simulink model "HOYAS_GRANDES_I"  (R2023b)
settings: Solver=FixedStepDiscrete  StartTime=0.0  StopTime=inf  FixedStep=Ts_Power  RelTol=1e-3  EnableMultiTasking=on
PostLoadFcn:
  | Ts_Power=50e-6;f=50;R_ac=0.12;L_ac=0.08/(2*pi*50);L1=0.17874;L2=0.07596;L3=0.04321;L4=0.01471;L5=0.04751;L6=0.2054;L7=0.17263;L8=0.14418;L9=0.17697;L10=0.19944;L11=0.18905;L12=0.26987;L13=0.1671;L14=0.16874;L15=0.14664;L16=0.12477;L17=0.14989;L18=0.17217;L19=0.19436; load('PV_prof_norm.mat');
InitFcn:
  | Ts_Power=50e-6;f=50;R_ac=0.12;L_ac=0.08/(2*pi*50);L1=0.17874;L2=0.07596;L3=0.04321;L4=0.01471;L5=0.04751;L6=0.2054;L7=0.17263;L8=0.14418;L9=0.17697;L10=0.19944;L11=0.18905;L12=0.26987;L13=0.1671;L14=0.16874;L15=0.14664;L16=0.12477;L17=0.14989;L18=0.17217;L19=0.19436; load('PV_prof_norm.mat');
undefined symbols (not defined in the file or in its folder): D11, Delta, L, X_ac
libraries: spsVoltageMeasurementLib x84, spsCurrentMeasurementLib x75, rtlab x41, spsThreePhaseSeriesRLCBranchLib x38, spsGroundLib x28, powerlib_extras x25, spsThreePhaseDynamicLoadLib x19, eeGeneralControl x4, rteventslib x4, spsThreePhasePISectionLineLib x2, spsThreePhaseTransformerTwoWindingsLib x2, spsPLLLib x1
(part 4 of 4)

== system HOYAS_GRANDES_I/SM_Computation/HOYAS GRANDES CT02/HG.1_CT.2-INV.08/Subsystem1 ==
  Current Measurement : spsCurrentMeasurementLib/Current Measurement  PhasorSimulation=off  OutputType=Complex  PSBequivalent=0
  Current Measurement1 : spsCurrentMeasurementLib/Current Measurement  PhasorSimulation=off  OutputType=Complex  PSBequivalent=0
  Current Measurement2 : spsCurrentMeasurementLib/Current Measurement  PhasorSimulation=off  OutputType=Complex  PSBequivalent=0
  Mux : Mux  Inputs=3
  a : PMIOPort  Side=Right
  ia : PMIOPort  Port=2  Side=Left
  ib : PMIOPort  Port=3  Side=Left
  b : PMIOPort  Port=4  Side=Right
  ic : PMIOPort  Port=5  Side=Left
  c : PMIOPort  Port=6  Side=Right
  i : Outport
  wires:
  Current Measurement1/1 -> Mux/2
  Current Measurement2/1 -> Mux/3
  Current Measurement/1 -> Mux/1
  Mux/1 -> i/1
  connections:
  ic/RConn1 -- Current Measurement2/LConn1
  ia/RConn1 -- Current Measurement/LConn1
  Current Measurement1/LConn1 -- ib/RConn1
  Current Measurement2/RConn1 -- c/RConn1
  Current Measurement/RConn1 -- a/RConn1
  Current Measurement1/RConn1 -- b/RConn1

== system HOYAS_GRANDES_I/SM_Computation/HOYAS GRANDES CT02/HG.1_CT.2-INV.09/Subsystem ==
  Ground2 : spsGroundLib/Ground  LConnTagsString=a
  Mux1 : Mux  Inputs=3
  Voltage a : spsVoltageMeasurementLib/Voltage Measurement  PhasorSimulation=off  OutputType=Complex  PSBequivalent=0
  Voltage b : spsVoltageMeasurementLib/Voltage Measurement  PhasorSimulation=off  OutputType=Complex  PSBequivalent=0
  Voltage c : spsVoltageMeasurementLib/Voltage Measurement  PhasorSimulation=off  OutputType=Complex  PSBequivalent=0
  Va : PMIOPort  Side=Left
  Vb : PMIOPort  Port=2  Side=Left
  Vc : PMIOPort  Port=3  Side=Left
  Vabc : Outport
  wires:
  Voltage c/1 -> Mux1/3
  Voltage a/1 -> Mux1/1
  Mux1/1 -> Vabc/1
  Voltage b/1 -> Mux1/2
  connections:
  Voltage c/LConn1 -- Vc/RConn1
  Voltage a/LConn1 -- Va/RConn1
  Voltage a/LConn2 -- Voltage b/LConn2 -- Voltage c/LConn2 -- Ground2/LConn1
  Voltage b/LConn1 -- Vb/RConn1

== system HOYAS_GRANDES_I/SM_Computation/HOYAS GRANDES CT02/HG.1_CT.2-INV.09/Subsystem1 ==
  Current Measurement : spsCurrentMeasurementLib/Current Measurement  PhasorSimulation=off  OutputType=Complex  PSBequivalent=0
  Current Measurement1 : spsCurrentMeasurementLib/Current Measurement  PhasorSimulation=off  OutputType=Complex  PSBequivalent=0
  Current Measurement2 : spsCurrentMeasurementLib/Current Measurement  PhasorSimulation=off  OutputType=Complex  PSBequivalent=0
  Mux : Mux  Inputs=3
  a : PMIOPort  Side=Right
  ia : PMIOPort  Port=2  Side=Left
  ib : PMIOPort  Port=3  Side=Left
  b : PMIOPort  Port=4  Side=Right
  ic : PMIOPort  Port=5  Side=Left
  c : PMIOPort  Port=6  Side=Right
  i : Outport
  wires:
  Mux/1 -> i/1
  Current Measurement/1 -> Mux/1
  Current Measurement2/1 -> Mux/3
  Current Measurement1/1 -> Mux/2
  connections:
  Current Measurement1/RConn1 -- b/RConn1
  Current Measurement/RConn1 -- a/RConn1
  Current Measurement2/RConn1 -- c/RConn1
  Current Measurement1/LConn1 -- ib/RConn1
  ia/RConn1 -- Current Measurement/LConn1
  ic/RConn1 -- Current Measurement2/LConn1

== system HOYAS_GRANDES_I/SM_Computation/HOYAS GRANDES CT02/Medidor18/Subsystem ==
  Ground2 : spsGroundLib/Ground  LConnTagsString=a
  Mux1 : Mux  Inputs=3
  Voltage a : spsVoltageMeasurementLib/Voltage Measurement  PhasorSimulation=off  OutputType=Complex  PSBequivalent=0
  Voltage b : spsVoltageMeasurementLib/Voltage Measurement  PhasorSimulation=off  OutputType=Complex  PSBequivalent=0
  Voltage c : spsVoltageMeasurementLib/Voltage Measurement  PhasorSimulation=off  OutputType=Complex  PSBequivalent=0
  Va : PMIOPort  Side=Left
  Vb : PMIOPort  Port=2  Side=Left
  Vc : PMIOPort  Port=3  Side=Left
  Vabc : Outport
  wires:
  Voltage c/1 -> Mux1/3
  Voltage a/1 -> Mux1/1
  Mux1/1 -> Vabc/1
  Voltage b/1 -> Mux1/2
  connections:
  Voltage c/LConn1 -- Vc/RConn1
  Voltage a/LConn1 -- Va/RConn1
  Voltage a/LConn2 -- Voltage b/LConn2 -- Voltage c/LConn2 -- Ground2/LConn1
  Voltage b/LConn1 -- Vb/RConn1

== system HOYAS_GRANDES_I/SM_Computation/HOYAS GRANDES CT02/Medidor18/Subsystem1 ==
  Current Measurement : spsCurrentMeasurementLib/Current Measurement  PhasorSimulation=off  OutputType=Complex  PSBequivalent=0
  Current Measurement1 : spsCurrentMeasurementLib/Current Measurement  PhasorSimulation=off  OutputType=Complex  PSBequivalent=0
  Current Measurement2 : spsCurrentMeasurementLib/Current Measurement  PhasorSimulation=off  OutputType=Complex  PSBequivalent=0
  Mux : Mux  Inputs=3
  a : PMIOPort  Side=Right
  ia : PMIOPort  Port=2  Side=Left
  ib : PMIOPort  Port=3  Side=Left
  b : PMIOPort  Port=4  Side=Right
  ic : PMIOPort  Port=5  Side=Left
  c : PMIOPort  Port=6  Side=Right
  i : Outport
  wires:
  Mux/1 -> i/1
  Current Measurement/1 -> Mux/1
  Current Measurement2/1 -> Mux/3
  Current Measurement1/1 -> Mux/2
  connections:
  Current Measurement1/RConn1 -- b/RConn1
  Current Measurement/RConn1 -- a/RConn1
  Current Measurement2/RConn1 -- c/RConn1
  Current Measurement1/LConn1 -- ib/RConn1
  ia/RConn1 -- Current Measurement/LConn1
  ic/RConn1 -- Current Measurement2/LConn1

== matlab function HOYAS_GRANDES_I/SM_Computation/MATLAB Function ==
  data: P_profile input; P output; P_ref input
function P = fcn(P_profile,P_ref)

if(P_profile>P_ref)
    P=P_ref;
else
    P=P_profile;
end
